simulink model "Total_Pjt"  (R2023b)
settings: Solver=FixedStepDiscrete  StartTime=0.0  StopTime=10.0  FixedStep=Ts  RelTol=1e-3
values from neighbouring files (symbols this model uses):
  Ts = 0.01    [para.m]
settings Model: Creator=User  LastModifiedBy=User
settings OptimizationCC: DefaultParameterBehavior=Inlined  EnhancedBackFolding=on  PassReuseOutputArgsAs=Individual arguments  ZeroExternalMemoryAtStartup=off  ZeroInternalMemoryAtStartup=off  OptimizeBlockOrder=speed  DifferentSizesBufferReuse=on  OptimizationCustomize=off  EfficientTunableParamExpr=on
settings DebuggingCC: ParameterTunabilityLossMsg=error
settings HardwareCC: ProdBitPerPointer=32  ProdBitPerSizeT=32  ProdBitPerPtrDiffT=32  ProdLargestAtomicFloat=None  ProdWordSize=32  ProdHWDeviceType=Infineon->TriCore
settings SFSimCC: MATLABDynamicMemAlloc=off
settings RTWCC: Description=Embedded Coder  SystemTargetFile=ert.tlc  GenCodeOnly=on  TemplateMakefile=ert_default_tmf
settings CodeAppCC: ForceParamTrailComments=on  IgnoreCustomStorageClasses=off  OperatorAnnotations=on  SimulinkDataObjDesc=on  SFDataObjDesc=on  InsertBlockDesc=on
settings ERTTargetCC: TargetLangStandard=C99 (ISO)  GenerateSampleERTMain=on  InlinedParameterPlacement=NonHierarchical  ERTCustomFileTemplate=example_file_process.tlc

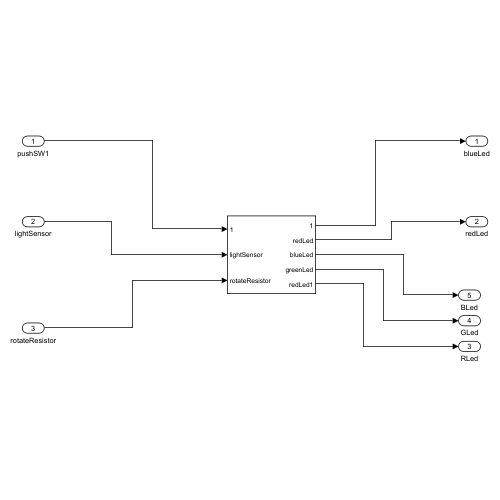
[thumbnail: Simulink's stored preview of the top-level diagram]
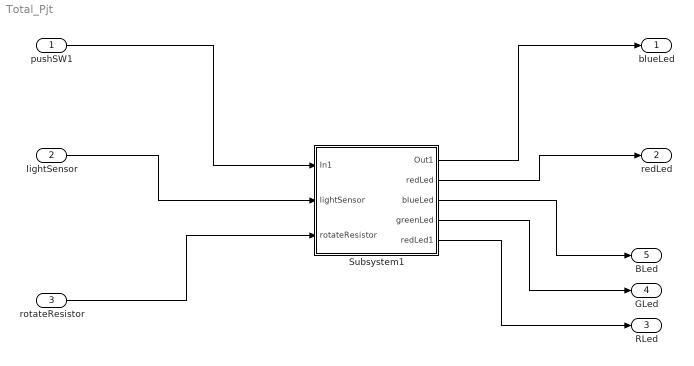
== system Total_Pjt ==
  pushSW1 : Inport  OutMin=0  OutMax=1  OutDataTypeStr=boolean
  lightSensor : Inport  Port=2  OutMin=0  OutMax=4096  OutDataTypeStr=uint16
  rotateResistor : Inport  Port=3  OutMin=0  OutMax=4096  OutDataTypeStr=uint16
  Subsystem1 : Subsystem
  blueLed : Outport  OutMin=0  OutMax=50000  OutDataTypeStr=uint16
  redLed : Outport  Port=2  OutMin=0  OutMax=50000  OutDataTypeStr=uint16
  RLed : Outport  Port=3  OutMin=0  OutMax=1  OutDataTypeStr=boolean
  GLed : Outport  Port=4  OutMin=0  OutMax=1  OutDataTypeStr=boolean
  BLed : Outport  Port=5  OutMin=0  OutMax=1  OutDataTypeStr=boolean
  wires:
  pushSW1/1 -> Subsystem1/1(In1)
  lightSensor/1 -> Subsystem1/2(lightSensor)
  rotateResistor/1 -> Subsystem1/3(rotateResistor)
  Subsystem1/1(Out1) -> blueLed/1
  Subsystem1/2(redLed) -> redLed/1
  Subsystem1/3(blueLed) -> BLed/1
  Subsystem1/4(greenLed) -> GLed/1
  Subsystem1/5(redLed1) -> RLed/1

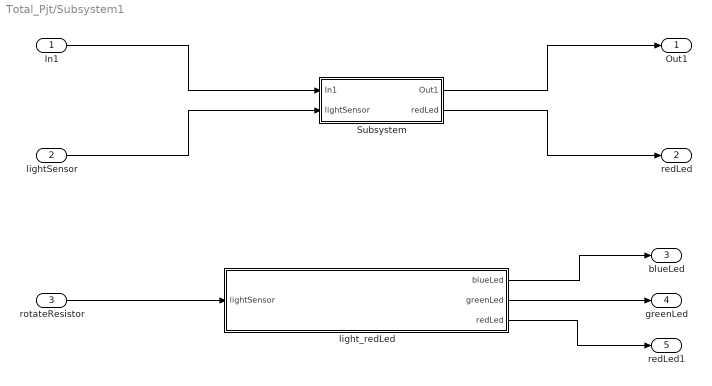
== system Total_Pjt/Subsystem1 ==
  In1 : Inport
  lightSensor : Inport  Port=2
  rotateResistor : Inport  Port=3
  Subsystem : Subsystem
  light_redLed : Subsystem
  Out1 : Outport
  redLed : Outport  Port=2
  blueLed : Outport  Port=3  OutDataTypeStr=boolean
  greenLed : Outport  Port=4  OutDataTypeStr=boolean
  redLed1 : Outport  Port=5  OutDataTypeStr=boolean
  wires:
  Subsystem/2(redLed) -> redLed/1
  Subsystem/1(Out1) -> Out1/1
  In1/1 -> Subsystem/1(In1)
  light_redLed/2(greenLed) -> greenLed/1
  lightSensor/1 -> Subsystem/2(lightSensor)
  light_redLed/3(redLed) -> redLed1/1
  rotateResistor/1 -> light_redLed/1(lightSensor)
  light_redLed/1(blueLed) -> blueLed/1

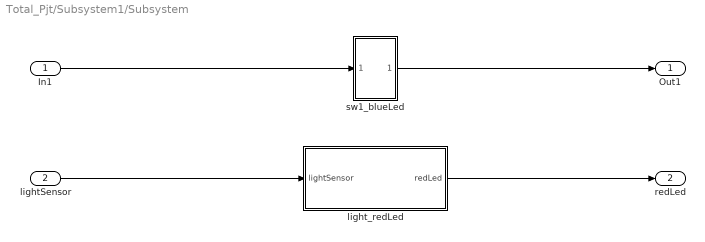
== system Total_Pjt/Subsystem1/Subsystem ==
  In1 : Inport
  lightSensor : Inport  Port=2
  light_redLed : Subsystem
  sw1_blueLed : Subsystem
  Out1 : Outport
  redLed : Outport  Port=2
  wires:
  light_redLed/1(redLed) -> redLed/1
  sw1_blueLed/1(Out1) -> Out1/1
  lightSensor/1 -> light_redLed/1(lightSensor)
  In1/1 -> sw1_blueLed/1(In1)

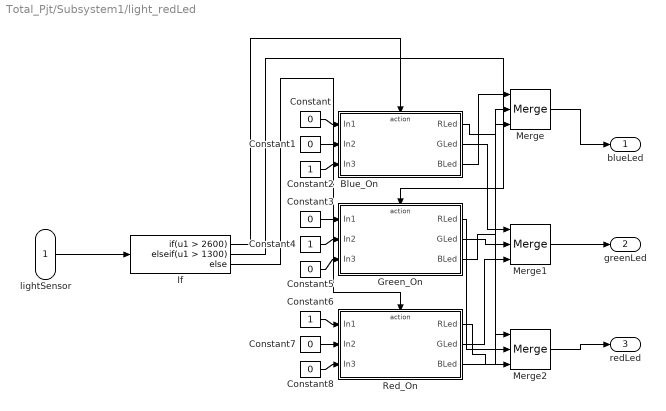
== system Total_Pjt/Subsystem1/light_redLed ==
  lightSensor : Inport
  Blue_On : Subsystem  TreatAsAtomicUnit=on
  Constant{,1,3,5,7..8} (6 alike) : Constant  Value=0  OutDataTypeStr=boolean
  Constant2 : Constant  OutDataTypeStr=boolean
  Constant4 : Constant  OutDataTypeStr=boolean
  Constant6 : Constant  OutDataTypeStr=boolean
  Green_On : Subsystem  TreatAsAtomicUnit=on
  If : If  IfExpression=u1 > 2600  ElseIfExpressions=u1 > 1300
  Merge : Merge  Inputs=3
  Merge1 : Merge  Inputs=3
  Merge2 : Merge  Inputs=3
  Red_On : Subsystem  TreatAsAtomicUnit=on
  blueLed : Outport
  greenLed : Outport  Port=2
  redLed : Outport  Port=3  OutDataTypeStr=boolean
  wires:
  lightSensor/1 -> If/1
  If/1 -> Blue_On/Action
  If/2 -> Green_On/Action
  If/3 -> Red_On/Action
  Merge/1 -> blueLed/1
  Merge2/1 -> redLed/1
  Blue_On/1(RLed) -> Merge2/1
  Green_On/1(RLed) -> Merge2/2
  Red_On/1(RLed) -> Merge2/3
  Merge1/1 -> greenLed/1
  Green_On/2(GLed) -> Merge1/2
  Red_On/2(GLed) -> Merge1/3
  Blue_On/2(GLed) -> Merge1/1
  Red_On/3(BLed) -> Merge/3
  Green_On/3(BLed) -> Merge/2
  Blue_On/3(BLed) -> Merge/1
  Constant/1 -> Blue_On/1(In1)
  Constant1/1 -> Blue_On/2(In2)
  Constant2/1 -> Blue_On/3(In3)
  Constant4/1 -> Green_On/2(In2)
  Constant5/1 -> Green_On/3(In3)
  Constant3/1 -> Green_On/1(In1)
  Constant7/1 -> Red_On/2(In2)
  Constant8/1 -> Red_On/3(In3)
  Constant6/1 -> Red_On/1(In1)

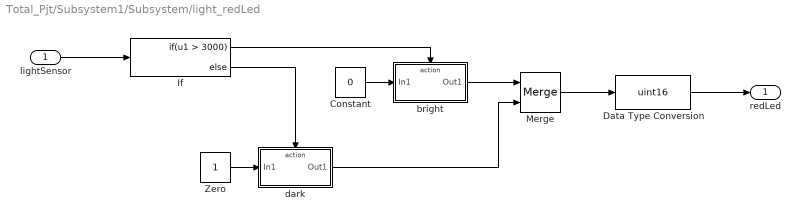
== system Total_Pjt/Subsystem1/Subsystem/light_redLed ==
  lightSensor : Inport
  Constant : Constant  Value=0
  Data Type Conversion : DataTypeConversion  OutDataTypeStr=uint16  SaturateOnIntegerOverflow=off  RndMeth=Floor
  If : If  IfExpression=u1 > 3000
  Merge : Merge
  Zero : Constant  OutDataTypeStr=double
  bright : Subsystem  TreatAsAtomicUnit=on
  dark : Subsystem  TreatAsAtomicUnit=on
  redLed : Outport
  wires:
  Merge/1 -> Data Type Conversion/1
  Data Type Conversion/1 -> redLed/1
  If/2 -> dark/Action
  lightSensor/1 -> If/1
  dark/1(Out1) -> Merge/2
  bright/1(Out1) -> Merge/1
  Zero/1 -> dark/1(In1)
  Constant/1 -> bright/1(In1)
  If/1 -> bright/Action

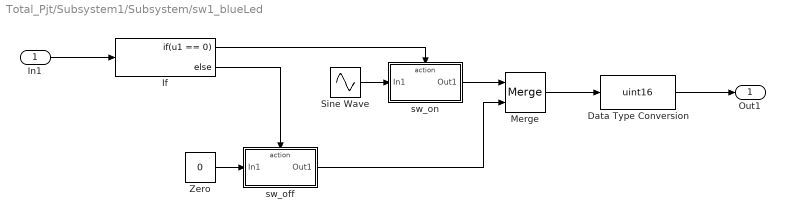
== system Total_Pjt/Subsystem1/Subsystem/sw1_blueLed ==
  In1 : Inport
  Data Type Conversion : DataTypeConversion  OutDataTypeStr=uint16  SaturateOnIntegerOverflow=off  RndMeth=Floor
  If : If  IfExpression=u1 == 0
  Merge : Merge
  Sine Wave : Sin  SineType=Sample based  Amplitude=25000  Bias=25000  Frequency=300  Samples=300  SampleTime=Ts
  Zero : Constant  Value=0  OutDataTypeStr=double
  sw_off : Subsystem  TreatAsAtomicUnit=on
  sw_on : Subsystem  TreatAsAtomicUnit=on
  Out1 : Outport  OutDataTypeStr=uint16
  wires:
  Merge/1 -> Data Type Conversion/1
  If/1 -> sw_on/Action
  Data Type Conversion/1 -> Out1/1
  If/2 -> sw_off/Action
  In1/1 -> If/1
  Sine Wave/1 -> sw_on/1(In1)
  sw_off/1(Out1) -> Merge/2
  sw_on/1(Out1) -> Merge/1
  Zero/1 -> sw_off/1(In1)

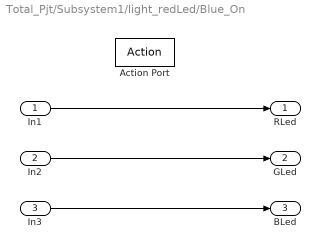
== system Total_Pjt/Subsystem1/light_redLed/Blue_On ==
  In1 : Inport
  In2 : Inport  Port=2
  In3 : Inport  Port=3
  Action Port : ActionPort  ActionPortLabel=if(u1 > 2600)
  RLed : Outport
  GLed : Outport  Port=2
  BLed : Outport  Port=3
  wires:
  In1/1 -> RLed/1
  In2/1 -> GLed/1
  In3/1 -> BLed/1

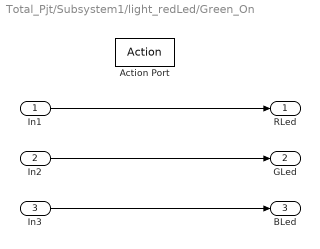
== system Total_Pjt/Subsystem1/light_redLed/Green_On ==
  In1 : Inport
  In2 : Inport  Port=2
  In3 : Inport  Port=3
  Action Port : ActionPort  ActionPortLabel=elseif(u1 > 1300)
  RLed : Outport
  GLed : Outport  Port=2
  BLed : Outport  Port=3
  wires:
  In1/1 -> RLed/1
  In2/1 -> GLed/1
  In3/1 -> BLed/1

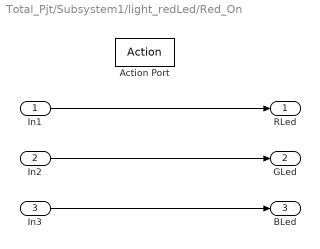
== system Total_Pjt/Subsystem1/light_redLed/Red_On ==
  In1 : Inport
  In2 : Inport  Port=2
  In3 : Inport  Port=3
  Action Port : ActionPort  ActionPortLabel=else
  RLed : Outport
  GLed : Outport  Port=2
  BLed : Outport  Port=3
  wires:
  In1/1 -> RLed/1
  In2/1 -> GLed/1
  In3/1 -> BLed/1

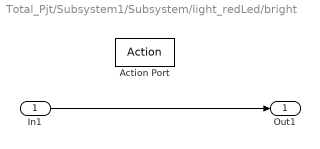
== system Total_Pjt/Subsystem1/Subsystem/light_redLed/bright ==
  In1 : Inport
  Action Port : ActionPort  ActionPortLabel=if(u1 > 3000)
  Out1 : Outport
  wires:
  In1/1 -> Out1/1

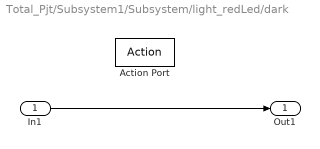
== system Total_Pjt/Subsystem1/Subsystem/light_redLed/dark ==
  In1 : Inport
  Action Port : ActionPort  ActionPortLabel=else
  Out1 : Outport
  wires:
  In1/1 -> Out1/1

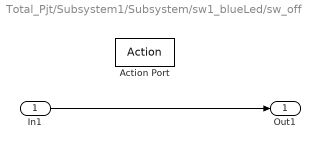
== system Total_Pjt/Subsystem1/Subsystem/sw1_blueLed/sw_off ==
  In1 : Inport
  Action Port : ActionPort  ActionPortLabel=else
  Out1 : Outport
  wires:
  In1/1 -> Out1/1

== system Total_Pjt/Subsystem1/Subsystem/sw1_blueLed/sw_on ==
  In1 : Inport
  Action Port : ActionPort  ActionPortLabel=if(u1 == 0)
  Out1 : Outport
  wires:
  In1/1 -> Out1/1
